simulink model "PlanerizerTest07_Flight_Stance"  (R2023a)
settings: Solver=FixedStepAuto  StartTime=0.0  StopTime=inf  FixedStep=0.005  RelTol=1e-3
libraries: canmsglib x8, speedgoatlib_IO691 x7, slrealtimeutilitieslib x3
settings Model: NumberOfSteps=2  ExtModeEnableFloating=off  Creator=celwe  LastModifiedBy=johna
settings SolverCC: ConcurrentTasks=on  PositivePriorityOrder=on
settings OptimizationCC: BlockReduction=off  OptimizeBlockIOStorage=off
settings DebuggingCC: TasksWithSamePriorityMsg=none  UnconnectedInputMsg=warning  UnconnectedOutputMsg=warning  UnconnectedLineMsg=warning
settings HardwareCC: ProdBitPerLong=64  ProdLongLongMode=on  ProdHWDeviceType=Intel->x86-64 (Linux 64)
settings ModelReferenceCC: EnableRefExpFcnMdlSchedulingChecks=on
settings RTWCC: Description=Simulink Real-Time  SystemTargetFile=slrealtime.tlc  TemplateMakefile=slrealtime_default_tmf  Toolchain=Simulink Real-Time Toolchain  BuildConfiguration=Faster Runs  CodeExecutionProfiling=on  TargetLang=C++  DLArmComputeVersion=19.05

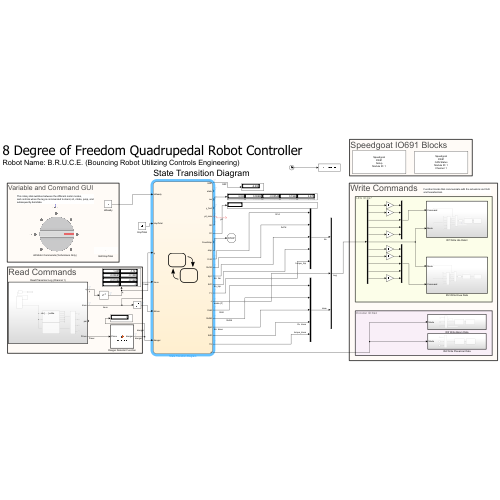
[thumbnail: Simulink's stored preview of the top-level diagram]
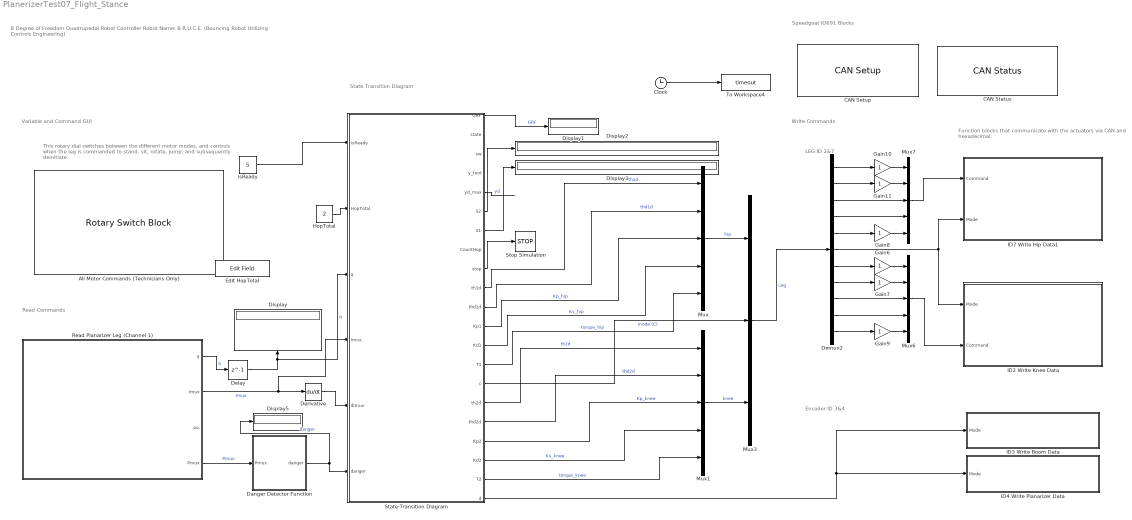
== system PlanerizerTest07_Flight_Stance ==
  note: Variable and Command GUI
  note: 8 Degree of Freedom Quadrupedal Robot Controller
      | Robot Name: B.R.U.C.E. (Bouncing Robot Utilizing Controls Engineering)
  note: This rotary dial switches between the different motor modes,
      | and controls when the leg is commanded to stand, sit, rotate, jump, and
      | subsequently deinitiate.
  note: LEG ID 2&7
  note: Function blocks that communicate with the actuators via CAN
      | and hexadecimal.
  note: Speedgoat IO691 Blocks
  note: Write Commands
  note: State Transition Diagram
  note: Encoder ID 3&4
  note: Read Commands
  "All Motor Commands (Technicians Only) " : RotarySwitchBlock
      settings: Values={{'Zeroing Planarizer', 'Zeroing Leg', 'Initiated', 'Control', 'deinit', 'Flight', 'test'}, [0 1 2 3 4 5 6]}
  "CAN Setup " : speedgoatlib_IO691/Legacy/CAN Setup   moduletype=IO691  id=1  pciSlot=-1  chn1=CAN (HS)  chn2=CAN (HS)  chn3=Disabled  chn4=Disabled  initStruct=[]  termStruct=[]  ArbitrationbdrChn1=1.0 MBaud  ArbitrationManbdrChn1=[2,8,31,8]  FdbdrChn1=5.0 MBaud  FdManbdrChn1=[2,2,5,2]  ArbitrationbdrChn2=1.0 MBaud  ArbitrationManbdrChn2=[2,8,31,8]  FdbdrChn2=5.0 MBaud  FdManbdrChn2=[2,2,5,2]  ArbitrationbdrChn3=1.0 MBaud  ArbitrationManbdrChn3=[2,8,31,8]  FdbdrChn3=5.0 MBaud  FdManbdrChn3=[2,2,5,2]  ArbitrationbdrChn4=1.0 MBaud  ArbitrationManbdrChn4=[2,8,31,8]  FdbdrChn4=5.0 MBaud  FdManbdrChn4=[2,2,5,2]  moduleInitValues=[691 1 -1 -1]
      settings: SourceProductName=Simulink Real-Time: Speedgoat I/O Blockset
  CAN Status : speedgoatlib_IO691/Legacy/CAN Status  moduleId=1  sampleTime=-1  channel=1  busRecovery=Off  arrayOutput=off  controllerCpuLoad=off  controllerLiveCount=off  initModeAct=off  avgBusLoad=off  receiving=off  RxQueueEmpty=off  dataOverrunRcv=off  rxBufferLevel=off  txPending=off  dataOverrunTx=off  txBufferLevel=off  errWarnLimit=off  errPassLimit=off  errBusOff=off  busRecoveryCounter=off  busCouplingErr=off  transceiverErr=off  opMode=off  brp=off  timeSegment1=off  timeSegment2=off  synchronisationJumpWidth=off  dataTSEG1=off  dataTSEG2=off  dataSJW=off  moduleType=691  qtyStatBlk=1  ptIdx=0  isFDMod=0
      settings: SourceProductName=Simulink Real-Time: Speedgoat I/O Blockset
  Clock : Clock
  Danger Detector Function : MATLAB Function  TreatAsAtomicUnit=on
  Delay : Delay  DelayLength=1
  Demux2 : Demux  Outputs=11
  Derivative : Derivative
  Display{,1..3,5} (5 alike) : Display
  Edit HopTotal : EditField  LabelPosition=Hide  ShowInitialText=on  Alignment=Center
  Gain{6..11} (6 alike) : Gain
  HopTotal : Constant  Value=2
  ID2 Write Knee Data : Subsystem  TreatAsAtomicUnit=on
  ID3 Write Boom Data : Subsystem  TreatAsAtomicUnit=on
  ID4 Write Planarizer Data : Subsystem  TreatAsAtomicUnit=on
  ID7 Write Hip Data1 : Subsystem  TreatAsAtomicUnit=on
  Mux{,1,6..7} (4 alike) : Mux  Inputs=5
  Mux3 : Mux  Inputs=3
  Read Planarizer Leg (Channel 1) : Subsystem  TreatAsAtomicUnit=on
  State-Transition Diagram : Stateflow chart  TreatAsAtomicUnit=on
      settings: PortSchema="{\"entries\":[{\"content\":{\"sides\":[{\"content\":{\"connectorIds\":[\"In3\",\"In5\",\"In1\",\"In6\",\"In4\",\"In2\"]},\"type\":\"ConnectorPlacement.EquallySpacedRectSide\",\"uuid\":\"09499f21-f50c-4ce4-914e-8b9942bcc246\"},{\"content\":{\"connectorIds\":[\"Out14\",\"Out16\",\"Out17\",\"Out18\",\"Out19\",\"Out20\",\"Out21\",\"Out15\",\"Out1\",\"Out10\",\"Out12\",\"Out5\",\"Out7\",\"Out3\",\"Out2\",\"Out11\",\"Out13\",\"Out6\",\"Out8\",\"Out4\",\"Out9\"],\"side\":\"RIGHT\"},\"type\":\"ConnectorPlacement.EquallySpacedRectSide\",\"uuid\":\"b935e908-ace3-4dfb-ad6d-08dfed6ffdb3\"},{\"content\":{\"side\":\"TOP\"},\"type\":\"ConnectorPlacement.EquallySpacedRectSide\",\"uuid\":\"4cd7c5d6-1f1f-4a1f-84b4-9b198395645e\"}]},\"type\":\"ConnectorPlacement.EquallySpacedConnector\",\"uuid\":\"2dc6a8af-05a8-4f21-87ab-6863f156f450\"}],\"packageUris\":[\"http://schema.mathworks.com/mf0/Connector/R2020b\"],\"version\":\"1.0\"}"
  Stop Simulation : Stop
  To Workspace4 : ToWorkspace  VariableName=timeout  SampleTime=-1
  isReady : Constant  Value=5
  wires:
  Mux/1 -> Mux3/1  "hip"
  State-Transition Diagram/3(T1) -> Mux/5  "torque_hip"
  Mux1/1 -> Mux3/3  "knee"
  State-Transition Diagram/2(c) -> Mux3/2  "mode (C)"
  isReady/1 -> State-Transition Diagram/3(isReady)
  Clock/1 -> To Workspace4/1
  Mux3/1 -> Demux2/1  "Leg"
  Mux7/1 -> ID7 Write Hip Data1/1(Command)
  Mux6/1 -> ID2 Write Knee Data/2(Command)
  Demux2/6 -> ID2 Write Knee Data/1(Mode), ID7 Write Hip Data1/2(Mode)
  Demux2/3 -> Mux7/3
  Demux2/8 -> Gain7/1
  Demux2/5 -> Gain8/1
  Demux2/4 -> Mux7/4
  Demux2/9 -> Mux6/3
  Demux2/2 -> Gain11/1
  Demux2/10 -> Mux6/4
  Gain11/1 -> Mux7/2
  Gain10/1 -> Mux7/1
  Gain7/1 -> Mux6/2
  Demux2/11 -> Gain9/1
  Gain9/1 -> Mux6/5
  Gain8/1 -> Mux7/5
  Gain6/1 -> Mux6/1
  State-Transition Diagram/8(Kd2) -> Mux1/4  "Kv_knee"
  State-Transition Diagram/4(T2) -> Mux1/5  "torque_knee"
  Demux2/1 -> Gain10/1
  Demux2/7 -> Gain6/1
  State-Transition Diagram/10(th1d) -> Mux/1  "th1d"
  State-Transition Diagram/12(thd1d) -> Mux/2  "thd1d"
  State-Transition Diagram/7(Kd1) -> Mux/4  "Kv_hip"
  State-Transition Diagram/5(Kp1) -> Mux/3  "Kp_hip"
  State-Transition Diagram/11(th2d) -> Mux1/1  "th2d"
  State-Transition Diagram/13(thd2d) -> Mux1/2  "thd2d"
  State-Transition Diagram/6(Kp2) -> Mux1/3  "Kp_knee"
  State-Transition Diagram/9(d) -> ID3 Write Boom Data/1(Mode), ID4 Write Planarizer Data/1(Mode)
  State-Transition Diagram/1(stop) -> Stop Simulation/1
  State-Transition Diagram/14(GRF) -> Display1/1  "GRF"
  Read Planarizer Leg (Channel 1)/2(Imux) -> State-Transition Diagram/6(Imux), Derivative/1  "Imux"
  Read Planarizer Leg (Channel 1)/1(q) -> Delay/1  "q"
  Delay/1 -> State-Transition Diagram/1(q), Display/1  "q"
  Danger Detector Function/1(danger) -> Display5/1, State-Transition Diagram/2(danger)  "danger"
  Derivative/1 -> State-Transition Diagram/4(dImux)
  Read Planarizer Leg (Channel 1)/4(Pmux) -> Danger Detector Function/1(Pmux)  "Pmux"
  HopTotal/1 -> State-Transition Diagram/5(HopTotal)
  State-Transition Diagram/19(yd_max) -> ?  "yd"
  State-Transition Diagram/20(S2) -> Display2/1
  State-Transition Diagram/21(S1) -> Display3/1

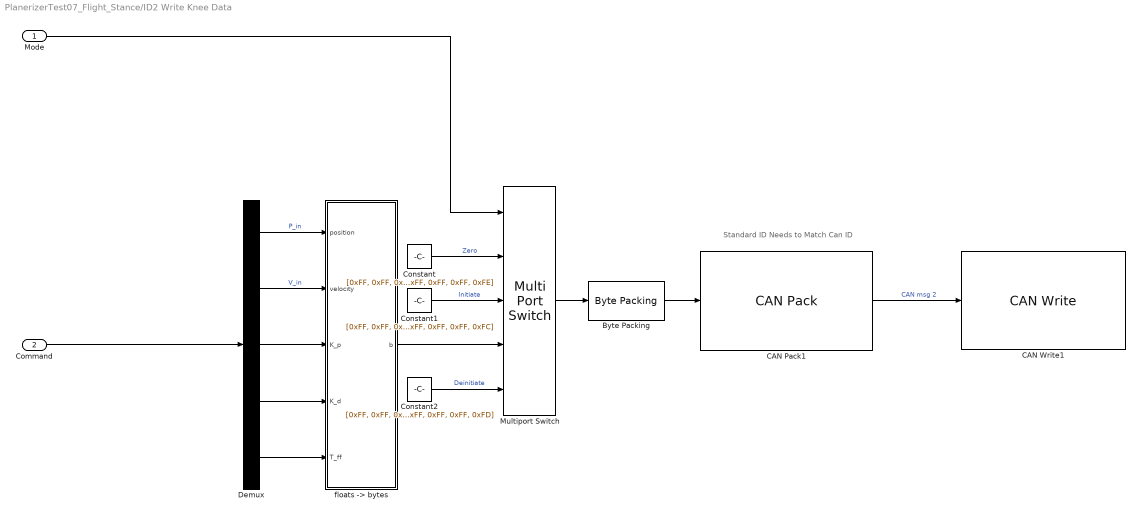
== system PlanerizerTest07_Flight_Stance/ID2 Write Knee Data ==
  note: Standard ID Needs to Match Can ID
  Mode : Inport
  Command : Inport  Port=2
  Byte Packing : slrealtimeutilitieslib/Byte Packing  MaskPackedDataType=uint8  MaskUnpackedDataTypes={['uint8']}  MaskAlignment=1
  CAN Pack1 : canmsglib/CAN Pack  MsgList=(none)  MsgName=CAN Msg  MsgIDType=Standard (11-bit identifier)  MsgIdentifier=2  MsgLength=8  Remote=off  ApplyMinMax=off  BusOutput=off  SignalInfo={ 'b1', '0', '8', 'LE', 'unsigned', 'Standard', '0', '1', '0', '-Inf', 'Inf'; 'b2', '8', '8', 'LE', 'unsigned', 'Standard', '0', '1', '0', '-Inf', 'Inf'; 'b3', '16', '8', 'LE', 'unsigned', 'Standard', '0', '1', '0', '-Inf', 'Inf'; 'b4', '24', '8', 'LE', 'unsigned', 'Standard', '0', '1', '0', '-Inf', 'Inf'; 'b5', '32', '8', 'LE', 'unsigned', 'Standard', '0', '1', '0', '-Inf', 'Inf'; 'b6', '40', '8', 'LE', 'unsigned', 'Standard', '0', '1', '0', '-Inf', 'Inf'; 'b7', '48', '8', 'LE', 'unsigned', 'Standard', '0', '1', '0', '-Inf', 'Inf'; 'b8', '56', '8', 'LE', 'unsigned', 'Standard', '0', '1', '0', '-Inf', 'Inf' }
      settings: DataFormat=raw data
  CAN Write1 : speedgoatlib_IO691/Legacy/CAN Write  id=1  ts=-1  channel=1  messageType=CAN  BusInput=off  enableStatusPort=off  canType=CAN (HS)  initValues=[691 1 -1 0 1 1 0 0]
      settings: SourceProductName=Simulink Real-Time: Speedgoat I/O Blockset
  Constant : Constant  Value=[0xFF, 0xFF, 0xFF, 0xFF, 0xFF, 0xFF, 0xFF, 0xFE]
  Constant1 : Constant  Value=[0xFF, 0xFF, 0xFF, 0xFF, 0xFF, 0xFF, 0xFF, 0xFC]
  Constant2 : Constant  Value=[0xFF, 0xFF, 0xFF, 0xFF, 0xFF, 0xFF, 0xFF, 0xFD]
  Demux : Demux  Outputs=5
  Multiport Switch : MultiPortSwitch  Inputs=4  DiagnosticForDefault=None  SaturateOnIntegerOverflow=off  InputSameDT=off
  "floats -> bytes" : MATLAB Function  TreatAsAtomicUnit=on
  wires:
  Demux/5 -> "floats -> bytes"/5(T_ff)
  Multiport Switch/1 -> Byte Packing/1
  Demux/4 -> "floats -> bytes"/4(K_d)
  Demux/1 -> "floats -> bytes"/1(position)  "P_in"
  Constant/1 -> Multiport Switch/2  "Zero"
  Demux/2 -> "floats -> bytes"/2(velocity)  "V_in"
  Constant2/1 -> Multiport Switch/5  "Deinitiate"
  CAN Pack1/1 -> CAN Write1/1  "CAN msg 2"
  Byte Packing/1 -> CAN Pack1/1
  Constant1/1 -> Multiport Switch/3  "Initiate"
  "floats -> bytes"/1(b) -> Multiport Switch/4
  Demux/3 -> "floats -> bytes"/3(K_p)
  Mode/1 -> Multiport Switch/1
  Command/1 -> Demux/1

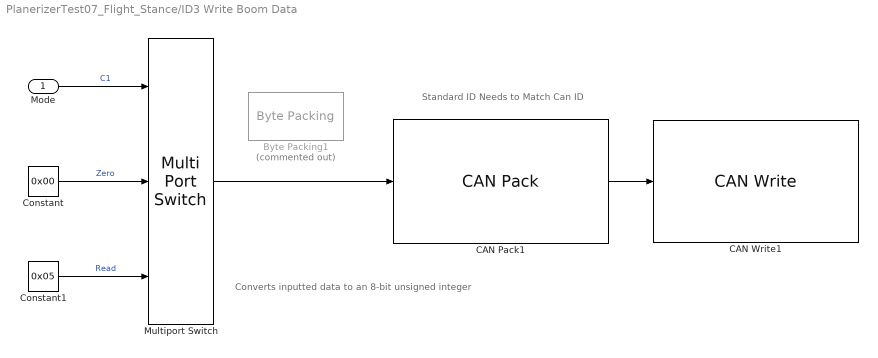
== system PlanerizerTest07_Flight_Stance/ID3 Write Boom Data ==
  note: Standard ID Needs to Match Can ID
  note: Converts inputted data to an 8-bit unsigned integer
  Mode : Inport
  Byte Packing1 : slrealtimeutilitieslib/Byte Packing  Commented=on  MaskPackedDataType=uint8  MaskUnpackedDataTypes={['uint8']}  MaskAlignment=1
  CAN Pack1 : canmsglib/CAN Pack  MsgList=(none)  MsgName=CAN Msg  MsgIDType=Standard (11-bit identifier)  MsgIdentifier=3  MsgLength=1  Remote=off  ApplyMinMax=off  BusOutput=off  SignalInfo={ 'b1', '0', '8', 'LE', 'unsigned', 'Standard', '0', '1', '0', '-Inf', 'Inf'; 'b2', '8', '8', 'LE', 'unsigned', 'Standard', '0', '1', '0', '-Inf', 'Inf'; 'b3', '16', '8', 'LE', 'unsigned', 'Standard', '0', '1', '0', '-Inf', 'Inf'; 'b4', '24', '8', 'LE', 'unsigned', 'Standard', '0', '1', '0', '-Inf', 'Inf'; 'b5', '32', '8', 'LE', 'unsigned', 'Standard', '0', '1', '0', '-Inf', 'Inf'; 'b6', '40', '8', 'LE', 'unsigned', 'Standard', '0', '1', '0', '-Inf', 'Inf'; 'b7', '48', '8', 'LE', 'unsigned', 'Standard', '0', '1', '0', '-Inf', 'Inf'; 'b8', '56', '8', 'LE', 'unsigned', 'Standard', '0', '1', '0', '-Inf', 'Inf' }
      settings: DataFormat=raw data
  CAN Write1 : speedgoatlib_IO691/Legacy/CAN Write  id=1  ts=-1  channel=1  messageType=CAN  BusInput=off  enableStatusPort=off  canType=CAN (HS)  initValues=[691 1 -1 0 1 1 0 0]
      settings: SourceProductName=Simulink Real-Time: Speedgoat I/O Blockset
  Constant : Constant  Value=0x00
  Constant1 : Constant  Value=0x05
  Multiport Switch : MultiPortSwitch  Inputs=2  DiagnosticForDefault=None  OutMin=0  SaturateOnIntegerOverflow=off  InputSameDT=off
  wires:
  Constant/1 -> Multiport Switch/2  "Zero"
  CAN Pack1/1 -> CAN Write1/1
  Multiport Switch/1 -> CAN Pack1/1
  Constant1/1 -> Multiport Switch/3  "Read"
  Mode/1 -> Multiport Switch/1  "C1"

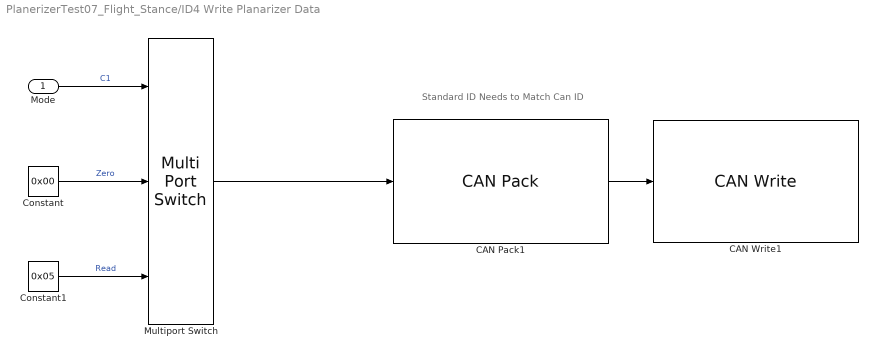
== system PlanerizerTest07_Flight_Stance/ID4 Write Planarizer Data ==
  note: Standard ID Needs to Match Can ID
  Mode : Inport
  CAN Pack1 : canmsglib/CAN Pack  MsgList=(none)  MsgName=CAN Msg  MsgIDType=Standard (11-bit identifier)  MsgIdentifier=4  MsgLength=1  Remote=off  ApplyMinMax=off  BusOutput=off  SignalInfo={ 'b1', '0', '8', 'LE', 'unsigned', 'Standard', '0', '1', '0', '-Inf', 'Inf'; 'b2', '8', '8', 'LE', 'unsigned', 'Standard', '0', '1', '0', '-Inf', 'Inf'; 'b3', '16', '8', 'LE', 'unsigned', 'Standard', '0', '1', '0', '-Inf', 'Inf'; 'b4', '24', '8', 'LE', 'unsigned', 'Standard', '0', '1', '0', '-Inf', 'Inf'; 'b5', '32', '8', 'LE', 'unsigned', 'Standard', '0', '1', '0', '-Inf', 'Inf'; 'b6', '40', '8', 'LE', 'unsigned', 'Standard', '0', '1', '0', '-Inf', 'Inf'; 'b7', '48', '8', 'LE', 'unsigned', 'Standard', '0', '1', '0', '-Inf', 'Inf'; 'b8', '56', '8', 'LE', 'unsigned', 'Standard', '0', '1', '0', '-Inf', 'Inf' }
      settings: DataFormat=raw data
  CAN Write1 : speedgoatlib_IO691/Legacy/CAN Write  id=1  ts=-1  channel=1  messageType=CAN  BusInput=off  enableStatusPort=off  canType=CAN (HS)  initValues=[691 1 -1 0 1 1 0 0]
      settings: SourceProductName=Simulink Real-Time: Speedgoat I/O Blockset
  Constant : Constant  Value=0x00
  Constant1 : Constant  Value=0x05
  Multiport Switch : MultiPortSwitch  Inputs=2  DiagnosticForDefault=None  SaturateOnIntegerOverflow=off  InputSameDT=off
  wires:
  Constant/1 -> Multiport Switch/2  "Zero"
  CAN Pack1/1 -> CAN Write1/1
  Multiport Switch/1 -> CAN Pack1/1
  Constant1/1 -> Multiport Switch/3  "Read"
  Mode/1 -> Multiport Switch/1  "C1"

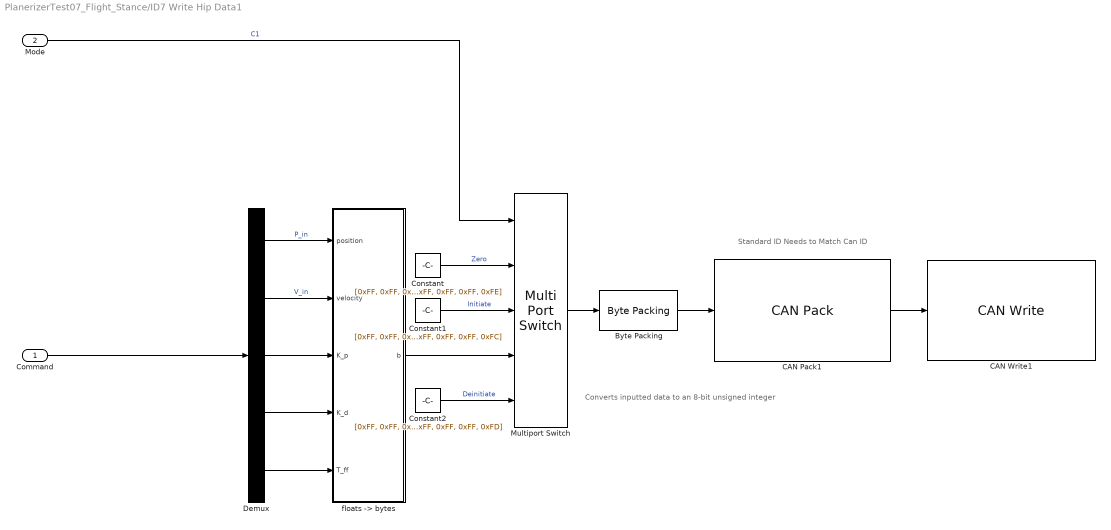
== system PlanerizerTest07_Flight_Stance/ID7 Write Hip Data1 ==
  note: Standard ID Needs to Match Can ID
  note: Converts inputted data to an 8-bit unsigned integer
  Command : Inport
  Mode : Inport  Port=2
  Byte Packing : slrealtimeutilitieslib/Byte Packing  MaskPackedDataType=uint8  MaskUnpackedDataTypes={['uint8']}  MaskAlignment=1
  CAN Pack1 : canmsglib/CAN Pack  MsgList=(none)  MsgName=CAN Msg  MsgIDType=Standard (11-bit identifier)  MsgIdentifier=7  MsgLength=8  Remote=off  ApplyMinMax=off  BusOutput=off  SignalInfo={ 'b1', '0', '8', 'LE', 'unsigned', 'Standard', '0', '1', '0', '-Inf', 'Inf'; 'b2', '8', '8', 'LE', 'unsigned', 'Standard', '0', '1', '0', '-Inf', 'Inf'; 'b3', '16', '8', 'LE', 'unsigned', 'Standard', '0', '1', '0', '-Inf', 'Inf'; 'b4', '24', '8', 'LE', 'unsigned', 'Standard', '0', '1', '0', '-Inf', 'Inf'; 'b5', '32', '8', 'LE', 'unsigned', 'Standard', '0', '1', '0', '-Inf', 'Inf'; 'b6', '40', '8', 'LE', 'unsigned', 'Standard', '0', '1', '0', '-Inf', 'Inf'; 'b7', '48', '8', 'LE', 'unsigned', 'Standard', '0', '1', '0', '-Inf', 'Inf'; 'b8', '56', '8', 'LE', 'unsigned', 'Standard', '0', '1', '0', '-Inf', 'Inf' }
      settings: DataFormat=raw data
  CAN Write1 : speedgoatlib_IO691/Legacy/CAN Write  id=1  ts=-1  channel=1  messageType=CAN  BusInput=off  enableStatusPort=off  canType=CAN (HS)  initValues=[691 1 -1 0 1 1 0 0]
      settings: SourceProductName=Simulink Real-Time: Speedgoat I/O Blockset
  Constant : Constant  Value=[0xFF, 0xFF, 0xFF, 0xFF, 0xFF, 0xFF, 0xFF, 0xFE]
  Constant1 : Constant  Value=[0xFF, 0xFF, 0xFF, 0xFF, 0xFF, 0xFF, 0xFF, 0xFC]
  Constant2 : Constant  Value=[0xFF, 0xFF, 0xFF, 0xFF, 0xFF, 0xFF, 0xFF, 0xFD]
  Demux : Demux  Outputs=5
  Multiport Switch : MultiPortSwitch  Inputs=4  DiagnosticForDefault=None  SaturateOnIntegerOverflow=off  InputSameDT=off
  "floats -> bytes" : MATLAB Function  TreatAsAtomicUnit=on
  wires:
  Demux/5 -> "floats -> bytes"/5(T_ff)
  Multiport Switch/1 -> Byte Packing/1
  Demux/4 -> "floats -> bytes"/4(K_d)
  Constant/1 -> Multiport Switch/2  "Zero"
  Demux/2 -> "floats -> bytes"/2(velocity)  "V_in"
  Constant2/1 -> Multiport Switch/5  "Deinitiate"
  CAN Pack1/1 -> CAN Write1/1
  Byte Packing/1 -> CAN Pack1/1
  Constant1/1 -> Multiport Switch/3  "Initiate"
  "floats -> bytes"/1(b) -> Multiport Switch/4
  Demux/3 -> "floats -> bytes"/3(K_p)
  Mode/1 -> Multiport Switch/1  "C1"
  Command/1 -> Demux/1
  Demux/1 -> "floats -> bytes"/1(position)  "P_in"

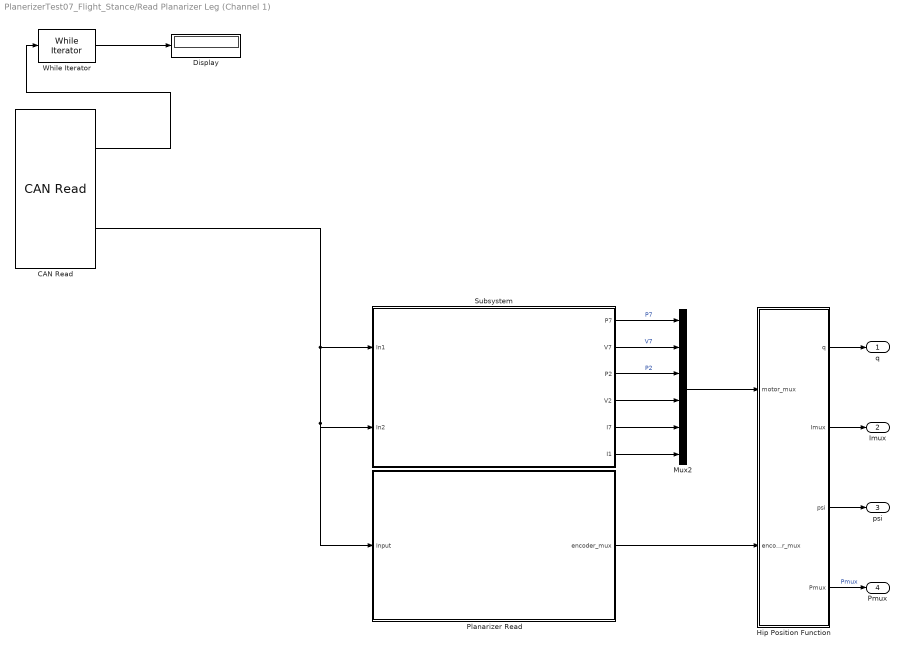
== system PlanerizerTest07_Flight_Stance/Read Planarizer Leg (Channel 1) ==
  CAN Read : speedgoatlib_IO691/Legacy/CAN Read  id=1  ts=-1  channel=1  messageType=CAN  canType=CAN (HS)  BusOutput=off  initValues=[691 1 -1 0 1 1 0]
      settings: SourceProductName=Simulink Real-Time: Speedgoat I/O Blockset
  Display : Display
  Hip Position Function : MATLAB Function  TreatAsAtomicUnit=on
  Mux2 : Mux  Inputs=6
  Planarizer Read : Subsystem
  Subsystem : Subsystem
  While Iterator : WhileIterator  MaxIters=-1  WhileBlockType=do-while  ResetStates=reset  ShowIterationPort=on
  q : Outport
  Imux : Outport  Port=2
  psi : Outport  Port=3
  Pmux : Outport  Port=4
  wires:
  CAN Read/1 -> While Iterator/1
  While Iterator/1 -> Display/1
  CAN Read/2 -> Planarizer Read/1(Input), Subsystem/2(In2), Subsystem/1(In1)
  Subsystem/1(P7) -> Mux2/1  "P7"
  Subsystem/3(P2) -> Mux2/3  "P2"
  Subsystem/2(V7) -> Mux2/2  "V7"
  Subsystem/4(V2) -> Mux2/4
  Planarizer Read/1(encoder_mux) -> Hip Position Function/2(encoder_mux)
  Mux2/1 -> Hip Position Function/1(motor_mux)
  Hip Position Function/1(q) -> q/1
  Hip Position Function/3(psi) -> psi/1
  Hip Position Function/4(Pmux) -> Pmux/1  "Pmux"
  Subsystem/5(I7) -> Mux2/5
  Subsystem/6(I1) -> Mux2/6
  Hip Position Function/2(Imux) -> Imux/1

== system PlanerizerTest07_Flight_Stance/Read Planarizer Leg (Channel 1)/Planarizer Read ==
  note: Encoder Read Command
  Input : Inport
  MATLAB Function : MATLAB Function  TreatAsAtomicUnit=on
  Mux : Mux
  Read Planarizer Leg (Chaannel 1) : Subsystem  TreatAsAtomicUnit=on
  encoder_mux : Outport
  wires:
  Read Planarizer Leg (Chaannel 1)/4(V4) -> Mux/4  "V4"
  Mux/1 -> MATLAB Function/1(in)
  Read Planarizer Leg (Chaannel 1)/1(P3) -> Mux/1  "P3"
  Read Planarizer Leg (Chaannel 1)/2(V3) -> Mux/2  "V3"
  Read Planarizer Leg (Chaannel 1)/3(P4) -> Mux/3  "P4"
  MATLAB Function/1(encoder_mux) -> encoder_mux/1
  Input/1 -> Read Planarizer Leg (Chaannel 1)/1(Input)

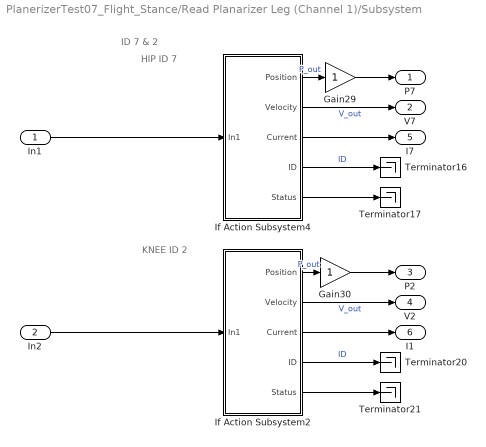
== system PlanerizerTest07_Flight_Stance/Read Planarizer Leg (Channel 1)/Subsystem ==
  note: KNEE ID 2
  note: HIP ID 7
  note: ID 7 & 2
  In1 : Inport
  In2 : Inport  Port=2
  Gain29 : Gain
  Gain30 : Gain
  If Action Subsystem2 : Subsystem  TreatAsAtomicUnit=on
  If Action Subsystem4 : Subsystem  TreatAsAtomicUnit=on
  Terminator{16..17,20..21} (4 alike) : Terminator
  P7 : Outport
  V7 : Outport  Port=2
  P2 : Outport  Port=3
  V2 : Outport  Port=4
  I7 : Outport  Port=5
  I1 : Outport  Port=6
  wires:
  If Action Subsystem4/4(ID) -> Terminator16/1  "ID"
  If Action Subsystem2/2(Velocity) -> V2/1  "V_out"
  If Action Subsystem2/5(Status) -> Terminator21/1
  If Action Subsystem4/2(Velocity) -> V7/1  "V_out"
  If Action Subsystem4/1(Position) -> Gain29/1  "P_out"
  If Action Subsystem4/3(Current) -> I7/1
  Gain30/1 -> P2/1
  If Action Subsystem2/4(ID) -> Terminator20/1  "ID"
  Gain29/1 -> P7/1
  If Action Subsystem4/5(Status) -> Terminator17/1
  If Action Subsystem2/1(Position) -> Gain30/1  "P_out"
  If Action Subsystem2/3(Current) -> I1/1
  In1/1 -> If Action Subsystem4/1(In1)
  In2/1 -> If Action Subsystem2/1(In1)

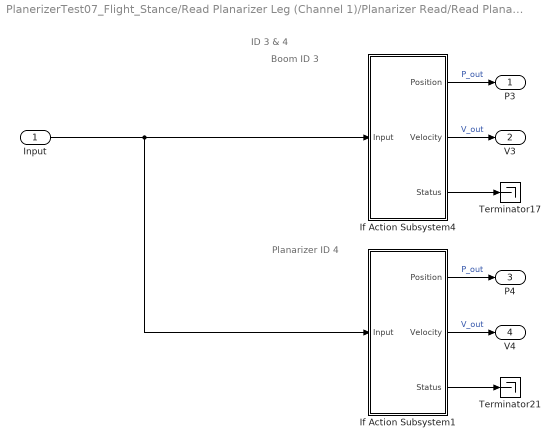
== system PlanerizerTest07_Flight_Stance/Read Planarizer Leg (Channel 1)/Planarizer Read/Read Planarizer Leg (Chaannel 1) ==
  note: Planarizer ID 4
  note: Boom ID 3
  note: ID 3 & 4
  Input : Inport
  If Action Subsystem1 : Subsystem  TreatAsAtomicUnit=on
  If Action Subsystem4 : Subsystem  TreatAsAtomicUnit=on
  Terminator17 : Terminator
  Terminator21 : Terminator
  P3 : Outport
  V3 : Outport  Port=2
  P4 : Outport  Port=3
  V4 : Outport  Port=4
  wires:
  If Action Subsystem1/1(Position) -> P4/1  "P_out"
  If Action Subsystem4/1(Position) -> P3/1  "P_out"
  If Action Subsystem4/3(Status) -> Terminator17/1
  If Action Subsystem1/2(Velocity) -> V4/1  "V_out"
  If Action Subsystem1/3(Status) -> Terminator21/1
  If Action Subsystem4/2(Velocity) -> V3/1  "V_out"
  Input/1 -> If Action Subsystem1/1(Input), If Action Subsystem4/1(Input)

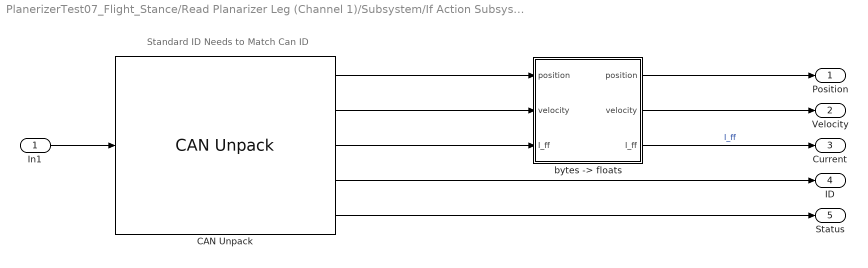
== system PlanerizerTest07_Flight_Stance/Read Planarizer Leg (Channel 1)/Subsystem/If Action Subsystem2 ==
  note: Standard ID Needs to Match Can ID
  In1 : Inport
  CAN Unpack : canmsglib/CAN Unpack  MsgList=(none)  MsgName=CAN Msg  MsgIDType=Standard (11-bit identifier)  MsgIdentifier=2  MsgLength=6  SignalInfo={ 'position', '16', '16', 'BE', 'unsigned', 'Standard', '0', '1', '0', '0', '65535'; 'velocity', '36', '12', 'BE', 'unsigned', 'Standard', '0', '1', '0', '0', '4095'; 'current', '40', '12', 'BE', 'unsigned', 'Standard', '0', '1', '0', '0', '4095'; 'id', '0', '8', 'BE', 'unsigned', 'Standard', '0', '1', '0', '0', '255' }  IDPort=off  TimestampPort=off  ErrorPort=off  RemotePort=off  LengthPort=off  StatusPort=on  ApplyMinMax=off
  "bytes -> floats" : MATLAB Function  TreatAsAtomicUnit=on
  Position : Outport
  Velocity : Outport  Port=2
  Current : Outport  Port=3
  ID : Outport  Port=4
  Status : Outport  Port=5
  wires:
  CAN Unpack/5 -> Status/1
  CAN Unpack/1 -> "bytes -> floats"/1("position ")
  CAN Unpack/3 -> "bytes -> floats"/3("I_ff ")
  "bytes -> floats"/1(position) -> Position/1
  CAN Unpack/4 -> ID/1
  "bytes -> floats"/2(velocity) -> Velocity/1
  "bytes -> floats"/3(I_ff) -> Current/1  "I_ff"
  CAN Unpack/2 -> "bytes -> floats"/2("velocity ")
  In1/1 -> CAN Unpack/1

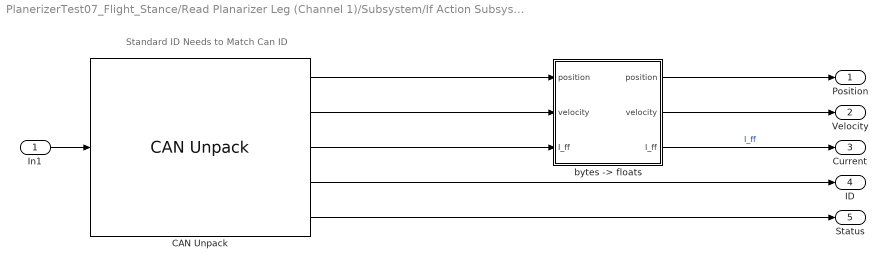
== system PlanerizerTest07_Flight_Stance/Read Planarizer Leg (Channel 1)/Subsystem/If Action Subsystem4 ==
  note: Standard ID Needs to Match Can ID
  In1 : Inport
  CAN Unpack : canmsglib/CAN Unpack  MsgList=(none)  MsgName=CAN Msg  MsgIDType=Standard (11-bit identifier)  MsgIdentifier=7  MsgLength=6  SignalInfo={ 'position', '16', '16', 'BE', 'unsigned', 'Standard', '0', '1', '0', '0', '65535'; 'velocity', '36', '12', 'BE', 'unsigned', 'Standard', '0', '1', '0', '0', '4095'; 'current', '40', '12', 'BE', 'unsigned', 'Standard', '0', '1', '0', '0', '4095'; 'id', '0', '8', 'BE', 'unsigned', 'Standard', '0', '1', '0', '0', '255' }  IDPort=off  TimestampPort=off  ErrorPort=off  RemotePort=off  LengthPort=off  StatusPort=on  ApplyMinMax=off
  "bytes -> floats" : MATLAB Function  TreatAsAtomicUnit=on
  Position : Outport
  Velocity : Outport  Port=2
  Current : Outport  Port=3
  ID : Outport  Port=4
  Status : Outport  Port=5
  wires:
  CAN Unpack/5 -> Status/1
  CAN Unpack/3 -> "bytes -> floats"/3("I_ff ")
  CAN Unpack/4 -> ID/1
  "bytes -> floats"/2(velocity) -> Velocity/1
  "bytes -> floats"/3(I_ff) -> Current/1  "I_ff"
  CAN Unpack/2 -> "bytes -> floats"/2("velocity ")
  In1/1 -> CAN Unpack/1
  CAN Unpack/1 -> "bytes -> floats"/1("position ")
  "bytes -> floats"/1(position) -> Position/1

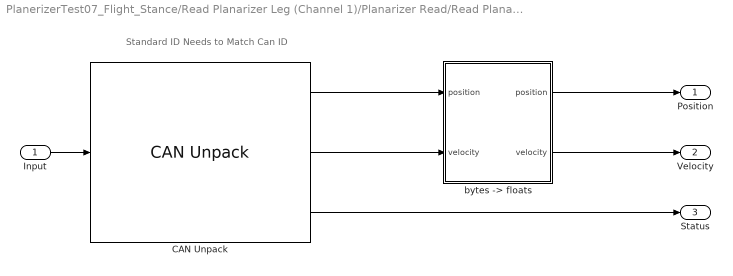
== system PlanerizerTest07_Flight_Stance/Read Planarizer Leg (Channel 1)/Planarizer Read/Read Planarizer Leg (Chaannel 1)/If Action Subsystem1 ==
  note: Standard ID Needs to Match Can ID
  Input : Inport
  CAN Unpack : canmsglib/CAN Unpack  MsgList=(none)  MsgName=CAN Msg  MsgIDType=Standard (11-bit identifier)  MsgIdentifier=4  MsgLength=6  SignalInfo={ 'position', '0', '32', 'LE', 'signed', 'Standard', '0', '1', '0', '0', '4294967295'; 'velocity', '32', '16', 'LE', 'signed', 'Standard', '0', '1', '0', '0', '65535' }  IDPort=off  TimestampPort=off  ErrorPort=off  RemotePort=off  LengthPort=off  StatusPort=on  ApplyMinMax=off
  "bytes -> floats" : MATLAB Function  TreatAsAtomicUnit=on
  Position : Outport
  Velocity : Outport  Port=2
  Status : Outport  Port=3
  wires:
  CAN Unpack/3 -> Status/1
  "bytes -> floats"/2(velocity) -> Velocity/1
  CAN Unpack/2 -> "bytes -> floats"/2("velocity ")
  Input/1 -> CAN Unpack/1
  CAN Unpack/1 -> "bytes -> floats"/1("position ")
  "bytes -> floats"/1(position) -> Position/1

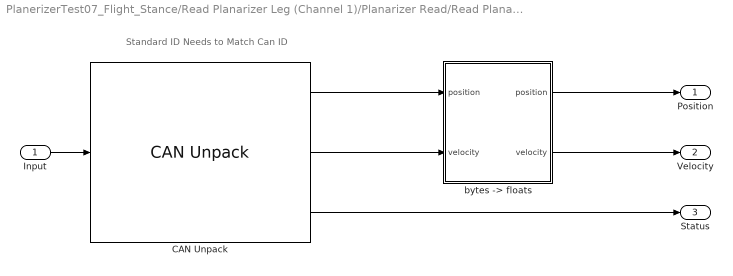
== system PlanerizerTest07_Flight_Stance/Read Planarizer Leg (Channel 1)/Planarizer Read/Read Planarizer Leg (Chaannel 1)/If Action Subsystem4 ==
  note: Standard ID Needs to Match Can ID
  Input : Inport
  CAN Unpack : canmsglib/CAN Unpack  MsgList=(none)  MsgName=CAN Msg  MsgIDType=Standard (11-bit identifier)  MsgIdentifier=3  MsgLength=6  SignalInfo={ 'position', '0', '32', 'LE', 'signed', 'Standard', '0', '1', '0', '0', '4294967295'; 'velocity', '32', '16', 'LE', 'signed', 'Standard', '0', '1', '0', '0', '65535' }  IDPort=off  TimestampPort=off  ErrorPort=off  RemotePort=off  LengthPort=off  StatusPort=on  ApplyMinMax=off
  "bytes -> floats" : MATLAB Function  TreatAsAtomicUnit=on
  Position : Outport
  Velocity : Outport  Port=2
  Status : Outport  Port=3
  wires:
  CAN Unpack/3 -> Status/1
  "bytes -> floats"/2(velocity) -> Velocity/1
  CAN Unpack/2 -> "bytes -> floats"/2("velocity ")
  Input/1 -> CAN Unpack/1
  CAN Unpack/1 -> "bytes -> floats"/1("position ")
  "bytes -> floats"/1(position) -> Position/1

== matlab function PlanerizerTest07_Flight_Stance/Read Planarizer Leg (Channel 1)/Subsystem/If Action Subsystem4/bytes -> floats ==
  data: position input; position output; velocity output; I_ff output; velocity input; I_ff input
function [position, velocity, I_ff] = fcn(position, velocity, I_ff)

P_MIN  =-95.5;  % [rad]
P_MAX  = 95.5;  % [rad]
V_MIN  =-45;    % [rad/s]
V_MAX  = 45;    % [rad/s]
I_MIN  =-40;    % []
I_MAX  = 40;    % []

position = position*(P_MAX  - P_MIN)/65535+ P_MIN;
velocity = velocity*(V_MAX  - V_MIN)/4095 + V_MIN;
I_ff     = I_ff*(I_MAX  - I_MIN)/4095 + I_MIN;

== matlab function PlanerizerTest07_Flight_Stance/Read Planarizer Leg (Channel 1)/Subsystem/If Action Subsystem2/bytes -> floats ==
  data: position input; position output; velocity output; I_ff output; velocity input; I_ff input
function [position, velocity, I_ff] = fcn(position, velocity, I_ff)

P_MIN  =-95.5;  % [rad]
P_MAX  = 95.5;  % [rad]
V_MIN  =-45;    % [rad/s]
V_MAX  = 45;    % [rad/s]
I_MIN  =-40;    % []
I_MAX  = 40;    % []

position = position*(P_MAX  - P_MIN)/65535+ P_MIN;
velocity = velocity*(V_MAX  - V_MIN)/4095 + V_MIN;
I_ff     = I_ff*(I_MAX  - I_MIN)/4095 + I_MIN;

== matlab function PlanerizerTest07_Flight_Stance/ID7 Write Hip Data1/floats -> bytes ==
  data: position input; b output uint8 size=8; velocity input; K_p input; K_d input; T_ff input
function b = fcn(position, velocity, K_p, K_d, T_ff)

P_MIN  =-95.5;  % [rad]
P_MAX  = 95.5;  % [rad]
V_MIN  =-45;    % [rad/s] 30 to 45
V_MAX  = 45;    % [rad/s]
KP_MIN = 0;     % [Nm/rad]
KP_MAX = 500;   % [Nm/rad]
KD_MIN = 0;     % [Nm*s/rad
KD_MAX = 5;     % [Nm*s/rad
T_MIN  =-18;    % [Nm]
T_MAX  = 18;    % [Nm]

position = floor((max(min(position,P_MAX) ,P_MIN)  - P_MIN )*65535/(P_MAX  - P_MIN));
velocity = floor((max(min(velocity,V_MAX) ,V_MIN)  - V_MIN )*4095 /(V_MAX  - V_MIN));
K_p      = floor((max(min(K_p     ,KP_MAX),KP_MIN) - KP_MIN)*4095 /(KP_MAX - KP_MIN));
K_d      = floor((max(min(K_d     ,V_MAX) ,V_MIN)  - KD_MIN)*4095 /(KD_MAX - KD_MIN));
T_ff     = floor((max(min(T_ff    ,V_MAX) ,V_MIN)  - T_MIN )*4095 /(T_MAX  - T_MIN));

p  = dec2bin(position);
p  = [repmat('0', 1, 16-length(p)),p];
v  = dec2bin(velocity);
v  = [repmat('0', 1, 12-length(v)),v];
kp = dec2bin(K_p);
kp  = [repmat('0', 1, 12-length(kp)),kp];
kd = dec2bin(K_d);
kd  = [repmat('0', 1, 12-length(kd)),kd];
t  = dec2bin(T_ff);
t  = [repmat('0', 1, 12-length(t)),t];

B = repmat('0', 8, 8);

B(1,:) = p(1:8);
B(2,:) = p(9:16);
B(3,:) = v(1:8);
B(4,:) = [v(9:12),kp(1:4)];
B(5,:) = kp(5:12);
B(6,:) = kd(1:8);
B(7,:) = [kd(9:12),t(1:4)];
B(8,:) = t(5:12);

B  = bin2dec(B);

b = uint8(B);

== matlab function PlanerizerTest07_Flight_Stance/Danger Detector Function ==
  data: Pmux input; danger output
function danger = isDanger(Pmux)
    % Pmux position matrix radians
    %       [p(ID1),p(ID2),p(ID3),p(IDN)]

        
    p1Max = 2; 
    p1Min = -2;
    p2Max = 2;
    p2Min = -2;
    
    P1 = Pmux(1:2:end);
    P2 = Pmux(2:2:end);
    
    danger = 0;
    if((0<sum((P1>p1Max) + (P1<p1Min))) || (0<sum((P2>p2Max) + (P2<p2Min))))
        danger = 1;
    end
end

== matlab function PlanerizerTest07_Flight_Stance/Read Planarizer Leg (Channel 1)/Planarizer Read/MATLAB Function ==
  data: in input; encoder_mux output
function encoder_mux = Pol2Cart(in)

% Variables
phi         = in(1);    % Boom Angle
phi_dot     = in(2);    % Boom Angular Velcoity
psi         = in(3);    % Planarizer Angle
psi_dot     = in(4);    % Planarizer Angular Velcoity

% Parameters
h           = .445;    % vertical height of base in meters
phi_offset  = .1995;        % Boom angle zero offset
b           = 1.2573;   % Length of boom to hip
e           = 0.137;    % horizantal length of encoders to mid-plane

% Outputs
x_hip = (e+b)*-psi;
x_dot_hip = (e+b)*-psi_dot;
y_hip = h - b*sin(phi+phi_offset);
y_dot_hip = - b*cos(phi+phi_offset)*phi_dot; 

encoder_mux = [x_hip x_dot_hip y_hip y_dot_hip psi];

== stateflow chart PlanerizerTest07_Flight_Stance/State-Transition Diagram ==
  state Start
  note: Simulink State Transition Diagram
      | "IsReady" is a user defined varable that controls the flow through the Finite State Mechine
      | Motor Commands: 1. Zero
      | (c) 2. Init
      | 3. Command
      | 4. Deinit
      | Encoder Commands: 1. Zero
      | (d) 2. Read
  state SlowDown
    entry:
    %deinitiate mode
    c = 4;
    d = 2;
  state ZeroPlanarizer
    entry:
    d = 1;
  state Init
    entry:
    c = 2;
    d = 2;
  state ZeroLeg
    entry:
    c = 1;
    to = 10;
  state Command
    entry:
    c = 3;
    tstep = 1.5;
    G = 1;
    n = 3;
    during:
    Tcalc1 = getT(Imux(1),q(1));
    Tcalc2 = getT(Imux(2),q(1)+q(2));
    [GRF,calcForceX] = getF(q,Tcalc1,Tcalc2);
    yd_filter  = AVGFilter(yd_filter,q(8),n);
    [y_foot,yd_foot] = getFootState(q,yd_filter);
    state Control [parallel]
      settings: executionOrder=1
      state ControllerSetup
        entry:
        %Flight
        sp = [.72 -1.15;0 0];
        Kp_f = [35,25];
        Kd_f = [50,10];
        F_offset = 1;
        %Stance
        w = 15*pi;
        Fxd = 0;
        yhipd = yhipCalc(sp,.5);
        Kp_s = [3; -3];
        Kdx_s = [-.12; .2];
        Kdy_s = [.05; -.1];
        % Temp Values
        Kp_temp = 30;
        Kd_temp = .2;
        %Goals
        th_LiftOff = deg2rad(65);
        Vxhipd = 1.5;
        offset = .5;
        Vyhipd = Vxhipd*tan(th_LiftOff);
      state Stand
        entry:
        state = 0;
        %Temp Gains
        Kp1 = Kp_temp;
        Kp2 = Kp_temp;
        Kd1 = Kd_temp;
        Kd2 = Kd_temp;
        %Stand Function
        to = t;
        th1d = q(1);
        tho1 = th1d;
        slope1 = (sp(1,1)*G - tho1)/tstep;
        th2d = q(2);
        tho2 = th2d;
        slope2 = (sp(1,2)*G - tho2)/tstep;
        during:
        th1d  = tho1  + slope1*(t-to);
        th2d  = tho2  + slope2*(t-to);
      state Ready2Jump
      state Airborn
        exit:
      state Stance
        during:
        T_ff = FeedForwardTorque(q,w,A,phi,Fxd,t-to);
        [T1, T2,S1,S2] = ControllerStance(q,Kp_s,Kdx_s,Kdy_s,T_ff,yhipd,Vxhipd,Vyhipd);
        exit:
        %Zeroing Torques
        T1 = 0;
        T2 = 0;
      state Transition2Stance
        entry:
        state = -2;
        to = t;
        %Stance Gains
        Kp1 = 0;
        Kp2 = 0;
        Kd1 = 0;
        Kd2 = 0;
        %Stance Transition
        [A,phi] = APhiGRFCalc(q,w,Vyhipd,GRF,F_offset)
      state Idle_Flight
        entry:
        state = 1
        idle = 0;
      state Flight
        during:
        [th1d,th2d,thd1d,thd2d] = Traj(t-to,tf,C);
        exit:
        % Zeroing Derivatives
        thd1d = 0;
        thd2d = 0;
        Kd1 = Kd_temp;
        Kd2 = Kd_temp;
      state Transition2Flight
        entry:
        state = 2;
        to = t;
        %Flight Gains
        Kp1 = Kp_f(1);
        Kp2 = Kp_f(2);
        Kd1 = Kd_f(1);
        Kd2 = Kd_f(2);
        %Flight Transition
        sp = Calc_Setpoint_Velcoity(q,sp,Vxhipd,offset);
        tf = FlightTimeApprox(y_max,yd_max,sp);
        C = TrajPlan(q,tf,sp);
        [th1d,th2d,thd1d,thd2d] = Traj(t-to,tf,C);
      state Idle_Stance
        entry:
        idle = 0;
      (default) -> ControllerSetup
      ControllerSetup -> Stand : {idle = 0;}
      Stand -> Ready2Jump : [(th1d >= sp(1,1)*G & slope1>0) | (th1d <= sp(1,1)*G & slope1<0)]
          | {th1d = sp(1,1)*G; th2d = sp(1,2)*G;}
      Ready2Jump -> Airborn : [isReady == 5 & sw == 0]
      Idle_Flight -> Stand [order 1] : [(isReady ~= 5 | CountHop >= HopTotal)]
      Airborn -> Transition2Stance : [after(2,sec)]
          | {CountHop = 0;}
      Idle_Flight -> Transition2Stance [order 2] : [sw == 0]
      Flight -> Idle_Flight : [after(tf,sec)]
      Transition2Stance -> Stance
      Transition2Flight -> Flight
      Idle_Stance -> Transition2Flight : [sw == 1]
      Stance -> Idle_Stance : [after(pi/w,sec)]
          | {CountHop = CountHop + 1;}
    state Detect [parallel]
      settings: executionOrder=2
      state Detect_Idle
        entry:
        idle = 1;
      state DetectImpact
        entry:
        I_lim =200*yd_max/.35;
        %I_sign1 = -q(1)/abs(q(1));
        %I_sign2 = -(q(1) + q(2))/abs(q(1) + q(2));
      state DetectLiftOff
        entry:
        yd_max = yd_filter;
      Detect_Idle -> DetectImpact [order 1] : [sw == 1 & idle == 0]
      DetectImpact -> Detect_Idle : [(abs(dImux(1)) > I_lim) | (abs(dImux(2)) > I_lim)]
          | {sw = 0;}
      (default) -> Detect_Idle : {sw = 1;}
      DetectLiftOff -> DetectLiftOff [order 2] : [yd_filter > yd_max]
      Detect_Idle -> DetectLiftOff [order 2] : [sw ==  0 & idle == 0]
      DetectLiftOff -> Detect_Idle [order 1] : [yd_max - yd_filter > .2]
          | {y_max = HipHeightAngleCalc(q); sw = 1;}
  state FinalShutdown
    entry:
    Kp1 = 0;
    Kp2 = 0;
    th1d = 0;
    th2d = 0;
    thd1d = 0;
    thd2d = 0;
    T1 = 0;
    T2 = 0;
    Kd1 = .1;
    Kd2 = .1;
  state Deinitiate
    entry:
    c = 4;
  (default) -> Start
  Start -> Init [order 2] : [isReady == 2]
  Start -> ZeroPlanarizer [order 1] : [isReady == 0 | isReady == 1]{to = 0;}
  SlowDown -> ZeroPlanarizer [order 2] : [after(.1,sec) & isReady == 0]
  ZeroPlanarizer -> SlowDown
  SlowDown -> Init [order 3] : [(isReady == 2 & to == 10) | isReady == 4]
  Init -> SlowDown [order 3] : [isReady == 0 | isReady == 1]
  Init -> FinalShutdown [order 2] : [isReady == 4 | danger == 1]
  Init -> Command [order 1] : [isReady == 3]
  ZeroLeg -> SlowDown
  SlowDown -> ZeroLeg [order 1] : [after(.5,sec) & isReady == 1 & ~(q(1) == q(2)) ]
  Command -> FinalShutdown : [isReady == 4 | danger == 1]
  FinalShutdown -> Deinitiate
  Deinitiate -> (junction 36) : after(3,sec)
  (junction 36) -> Deinitiate : {stop = 1;}
  data: YHIPD function_output; SP function_input; P function_input; A_Mag function_output; u function_input; W function_input; VYHIPD function_input; grf function_input; PHI function_output; OFFSET function_input; u function_input; SP function_output; SP function_input; VXHIPD function_input; OFFSET function_input; Y function_input; YD function_input; SP function_input; TF function_output; u function_input; TF function_input; SP function_input; C_mat function_output; TAU_ff function_output; u function_input; W function_input; A_Mag function_input; PHI function_input; FXD function_input; t function_input; t function_input; TF function_input; C_mat function_input; TH1D function_output; TH2D function_output; THD1D function_output; THD2D function_output; tau1 function_output double; u function_input; KP_s function_input; KDx_s function_input; KDy_s function_input; tau_ff function_input; YHIPd function_input; VXHIPd function_input; VYHIPd function_input; tau2 function_output; s1 function_output; s2 function_output; I function_input; CALC_T function_output; TH function_input; u function_input; T1CALC function_input; T2CALC function_input; calcFY function_output; calcFX function_output; in function_input; New function_input; out function_output; N function_input; u function_input; posy function_output; vely function_output; yd function_input; Y function_output; u function_input; q input; stop output =0; c output; T1 output =0; T2 output =0; Kp1 output =30; Kp2 output =30; Kd1 output =.2; Kd2 output =.2; danger input; isReady input; d output; th1d output =0; th2d output =0; thd1d output =0; thd2d output =0; Kd_f local; Kp_f local; Kp_s local; Vyhipd local; w local; Kd_temp local; Kp_temp local; Vxhipd local; to local; tho1 local; slope2 local; tho2 local; offset local; sp local; thd local; GRF output =0; calcForceX local; Tcalc1 local; Tcalc2 local; tstep local; slope1 local; th_LiftOff local; A local; CountHop output; Fxd local; T_ff local; phi local; yhipd local; tf local; C local; n local; G local; Kdx_s local; Kdy_s local; dImux input; state output; F_offset local; I_lim local; I_sign1 local; I_sign2 local; idle local; sw output; HopTotal input; yd_foot local; yd_filter local =0; y_foot output =0; y_max local; yd_max output; Imux input; S2 output; S1 output
  function YHIPD  = yhipCalc(SP,P):
    | function YHIPD  = yhipCalc(SP,P)
    | 
    |     % Length Constants
    |     LA = 0.1362;
    |     LB = 0.1636;
    | 
    |     YHIPD = (LB + LA)*(1-P) + (LA*cos(SP(1,1)) + LB*cos(SP(1,1)+SP(1,2)))*P;
    | end
  function [A_Mag,PHI] = APhiGRFCalc(u,W,VYHIPD,grf,OFFSET):
    | function [A_Mag,PHI] = APhiGRFCalc(u,W,VYHIPD,grf,OFFSET)
    | 
    |     % Mass Constants
    |     m0 = 0.665;
    |     m1 = 1.019;
    |     m2 = 0.128;
    |     % Length Constants
    |     LA = 0.1362;
    |     LB = 0.1636;
    | 
    | 
    |     %Actual hip velocity
    |     YD = u(5)*(-LB*sin(u(1)+u(2)) - LA*sin(u(1))) + u(6)*(-LB*sin(u(1)+u(2)));
    | 
    |     if grf > 800
    |         grf = 800;
    |     elseif grf < -800
    |         grf = -800;
    |     end
    |     
    |     A_Mag = OFFSET*(((m0+m1+m2)*W*(VYHIPD - YD))^2 + (grf)^2)/(2*(m0+m1+m2)*W*(VYHIPD - YD));
    |     PHI = asin(grf/A_Mag);
    | end
  function SP = Calc_Setpoint_Velcoity(u,SP,VXHIPD,OFFSET):
    | function SP = Calc_Setpoint_Velcoity(u,SP,VXHIPD,OFFSET)
    | 
    |     % Length Constants
    |     LA = 0.1362;
    |     LB = 0.1636;
    | 
    | 
    | 
    |     % CALC VX_FOOT
    |     VX_FOOT = u(7) + u(5)*LA*cos(u(1)) + (u(5)+ u(6))*LB*cos(u(1)+ u(2));
    | 
    |     % CALC NEW SETPOINT VELOCITY
    |     SP(2,1) = -2*(VXHIPD-VX_FOOT)*OFFSET/(LA*cos(SP(1,1)) + LB*cos(SP(1,1) + SP(1,2)));
    |     SP(2,2) = (VXHIPD-VX_FOOT)*OFFSET/(LB*cos(SP(1,1) + SP(1,2)));
    | end
  function TF = FlightTimeApprox(Y,YD,SP):
    | function TF = FlightTimeApprox(Y,YD,SP)
    | 
    |     % Mass Constants
    |     m0 = 0.665;
    |     m1 = 1.019;
    |     m2 = 0.128;
    |     % Length Constants
    |     LA = 0.1362;
    |     LB = 0.1636;
    |     L1 = 0.011;
    |     L2 = 0.0527;
    |     % Bar Mass Inertias
    |     I1 = 0.00207;
    |     I2 = 0.00191;
    |     % Damping Coefficents
    |     c1 = 0.00749;
    |     c2 = 1;
    |     % Gravity
    |     g = 7;
    | 
    |     yf = LA*cos(SP(1,1)) + LB*cos(SP(1,1)+SP(1,2));
    |     if((YD^2-2*g*(yf-Y))>=0)
    |         TF = (YD + sqrt(YD^2-2*g*(yf-Y)))/g;
    |     else
    |         TF = 0.005;
    |     end
    | end
  function C_mat = TrajPlan(u,TF,SP):
    | function C_mat = TrajPlan(u,TF,SP)
    | 
    |     M_t =[1   0    0    0;
    |           0   1    0    0;
    |           1   TF   TF^2 TF^3;
    |           0   1    2*TF 3*TF^2];
    | 
    |     M_IC = [u(1) u(2); u(5) u(6); SP];
    | 
    |     C_mat = M_t\M_IC;
    | end
  function TAU_ff  = FeedForwardTorque(u,W,A_Mag,PHI,FXD,t):
    | function TAU_ff  = FeedForwardTorque(u,W,A_Mag,PHI,FXD,t)
    | 
    |     % Mass Constants
    |     m0 = 0.665;
    |     m1 = 1.019;
    |     m2 = 0.128;
    |     % Length Constants
    |     LA = 0.1362;
    |     LB = 0.1636;
    |     L1 = 0.011;
    |     L2 = 0.0527;
    |     % Bar Mass Inertias
    |     I1 = 0.00207;
    |     I2 = 0.00191;
    |     % Damping Coefficents
    |     c1 = 0.00749;
    |     c2 = 1;
    |     % Gravity
    |     g = 9.81;
    | 
    |     Fd = [FXD; A_Mag*sin(W*t + PHI)];
    |     J = [LB*cos(u(1)+u(2)) + LA*cos(u(1))  LB*cos(u(1)+u(2));
    |         LB*sin(u(1)+u(2)) + LA*sin(u(1))  LB*sin(u(1)+u(2))];
    |     
    |     tau_mass = [m1*g*L1*sin(u(1)) + m2*g*(L2*sin(u(1)+u(2)) + LA*sin(u(1)));
    |               m2*g*L2*sin(u(1)+u(2))];
    |     TAU_ff = -J'*Fd + tau_mass;
    | end
  function [TH1D,TH2D,THD1D,THD2D] = Traj(t,TF,C_mat):
    | function [TH1D,TH2D,THD1D,THD2D] = Traj(t,TF,C_mat)
    | 
    |     if TF < t
    |         t = TF;
    |     end
    |     
    |     thd = [1 t   t^2 t^3;
    |            0 1 2*t 3*t^2]*C_mat;
    | 
    |     % Position th1d
    |     TH1D = thd(1,1);
    |     % Position th2d
    |     TH2D = thd(1,2);
    |     if TH2D < -1.8
    |         TH2D = -1.8;
    |     end
    |     % Position Derivative thd1d
    |     THD1D = thd(2,1);
    |     % Position Derivative thd2d
    |     THD2D = thd(2,2);
    | end
  function [tau1,tau2,s1,s2] = ControllerStance(u,KP_s,KDx_s,KDy_s,tau_ff,YHIPd,VXHIPd,VYHIPd):
    | function [tau1,tau2,s1,s2] = ControllerStance(u,KP_s,KDx_s,KDy_s,tau_ff,YHIPd,VXHIPd,VYHIPd)
    |     % Length Constants
    |     LA = 0.1362;
    |     LB = 0.1636;
    | 
    |     %Calculate Actual Values
    |     YHIPa = LB*cos(u(1)+u(2)) + LA*cos(u(1));
    |     VXHIPa = u(5)*(-LB*cos(u(1)+u(2)) - LA*cos(u(1))) + u(6)*(-LB*cos(u(1)+u(2)));
    |     VYHIPa = u(5)*(-LB*sin(u(1)+u(2)) - LA*sin(u(1))) + u(6)*(-LB*sin(u(1)+u(2)));
    | 
    |     % Hip y Position
    |     e_y = YHIPd - YHIPa;
    |     % Hip x Velecity
    |     e_Vx = VXHIPd - VXHIPa;
    |     % Hip y Velecity
    |     e_Vy = VYHIPd -VYHIPa;
    |     % Compute error Matricies
    | 
    |     T = tau_ff + KP_s*e_y + KDx_s*e_Vx + KDy_s*e_Vy;
    |     tau1 = T(1);
    |     tau2 = T(2);
    | 
    |     s1 = [tau_ff(1) KP_s(1)*e_y KDx_s(1)*e_Vx KDy_s(1)*e_Vy tau1];
    |     s2 = [tau_ff(2) KP_s(2)*e_y KDx_s(2)*e_Vx KDy_s(2)*e_Vy tau2];
    | end
  function CALC_T = getT(I,TH):
    | function CALC_T = getT(I,TH)
    |     CALC_T = I/abs(4.8*sin(TH));
    | end
  function [calcFY,calcFX] = getF(u,T1CALC,T2CALC):
    | function [calcFY,calcFX] = getF(u,T1CALC,T2CALC)
    | 
    |     % Length Constants
    |     LA = 0.1362;
    |     LB = 0.1636;
    | 
    | 
    |     J = [LB*cos(u(1)+u(2)) + LA*cos(u(1))  LB*cos(u(1)+u(2));
    |          LB*sin(u(1)+u(2)) + LA*sin(u(1))  LB*sin(u(1)+u(2))];
    |     %T_mass = [m1*g*L1*sin(u(1)) + m2*g*(L2*sin(u(1)+u(2)) + LA*sin(u(1)));
    |     %             m2*g*L2*sin(u(1)+u(2))]*0;
    | 
    |     T = [T1CALC;T2CALC];
    |     
    |     F = (-J')\(T); %check sign on T_mass
    | 
    |     calcFY = F(2);
    |     calcFX = F(1);
    | end
  function out  = AVGFilter(in,New,N):
    | function out  = AVGFilter(in,New,N)
    |     out = in*(N-1)/N+New/N;
    | end
  function [posy,vely]   = getFootState(u,yd):
    | function [posy,vely]   = getFootState(u,yd)
    |     % Length Constants
    |     LA = 0.1362;
    |     LB = 0.1636;
    | 
    |     r_foot = .055;
    | 
    | 
    |     x_foot = [u(3) + LA*sin(u(1)) + (LB-r_foot)*sin(u(1)+ u(2));
    |               u(4) - LA*cos(u(1)) - (LB-r_foot)*cos(u(1)+ u(2)) - r_foot];
    | 
    |     v_foot = [u(7) + u(5)*LA*cos(u(1)) + (u(5)+ u(6))*(LB-r_foot)*cos(u(1)+ u(2));
    |                 yd + u(5)*LA*sin(u(1)) + (u(5)+ u(6))*(LB-r_foot)*sin(u(1)+ u(2))];
    | 
    |     posy = x_foot(2);
    |     vely = v_foot(2);
    | end
  function Y   = HipHeightAngleCalc(u):
    | function Y   = HipHeightAngleCalc(u)
    |     % Length Constants
    |     LA = 0.1362;
    |     LB = 0.1636;
    | 
    | 
    |     Y = LB*cos(u(1)+u(2)) + LA*cos(u(1));
    |     %YD = u(5)*(-LB*sin(u(1)+u(2)) - LA*sin(u(1))) + u(6)*(-LB*sin(u(1)+u(2)));
    | end

== matlab function PlanerizerTest07_Flight_Stance/Read Planarizer Leg (Channel 1)/Hip Position Function ==
  data: q output; Imux output; psi output; motor_mux input; Pmux output; encoder_mux input
function [q,Imux,psi,Pmux] = Hip_Position(motor_mux,encoder_mux)
    q = [motor_mux(1),motor_mux(3),encoder_mux(1),encoder_mux(3),motor_mux(2),motor_mux(4),encoder_mux(2),encoder_mux(4)];
    Imux = [motor_mux(5),motor_mux(6)];
    psi = encoder_mux(5);
    Pmux = [motor_mux(1),motor_mux(3)];
end

== matlab function PlanerizerTest07_Flight_Stance/Read Planarizer Leg (Channel 1)/Planarizer Read/Read Planarizer Leg (Chaannel 1)/If Action Subsystem1/bytes -> floats ==
  data: position input; position output; velocity output; velocity input
function [position, velocity] = fcn(position, velocity)

CPR  = 40000;  % [Counts Per Revolution]
F    = 1000;   % [Samples Per Second]

position = position/CPR*(2*pi());
velocity = velocity/CPR*(2*pi())*F;

== matlab function PlanerizerTest07_Flight_Stance/Read Planarizer Leg (Channel 1)/Planarizer Read/Read Planarizer Leg (Chaannel 1)/If Action Subsystem4/bytes -> floats ==
  data: position input; position output; velocity output; velocity input
function [position, velocity] = fcn(position, velocity)

CPR  = 40000;  % [Counts Per Revolution]
F    = 1000;   % [Samples Per Second]

position = position/CPR*(2*pi());
velocity = velocity/CPR*(2*pi())*F;

== matlab function PlanerizerTest07_Flight_Stance/ID2 Write Knee Data/floats -> bytes ==
  data: position input; b output uint8 size=8; velocity input; K_p input; K_d input; T_ff input
function b = fcn(position, velocity, K_p, K_d, T_ff)

P_MIN  =-95.5;  % [rad]
P_MAX  = 95.5;  % [rad]
V_MIN  =-45;    % [rad/s] 30 to 45
V_MAX  = 45;    % [rad/s]
KP_MIN = 0;     % [Nm/rad]
KP_MAX = 500;   % [Nm/rad]
KD_MIN = 0;     % [Nm*s/rad
KD_MAX = 5;     % [Nm*s/rad
T_MIN  =-18;    % [Nm]
T_MAX  = 18;    % [Nm]

position = floor((max(min(position,P_MAX) ,P_MIN)  - P_MIN )*65535/(P_MAX  - P_MIN));
velocity = floor((max(min(velocity,V_MAX) ,V_MIN)  - V_MIN )*4095 /(V_MAX  - V_MIN));
K_p      = floor((max(min(K_p     ,KP_MAX),KP_MIN) - KP_MIN)*4095 /(KP_MAX - KP_MIN));
K_d      = floor((max(min(K_d     ,V_MAX) ,V_MIN)  - KD_MIN)*4095 /(KD_MAX - KD_MIN));
T_ff     = floor((max(min(T_ff    ,V_MAX) ,V_MIN)  - T_MIN )*4095 /(T_MAX  - T_MIN));

p  = dec2bin(position);
p  = [repmat('0', 1, 16-length(p)),p];
v  = dec2bin(velocity);
v  = [repmat('0', 1, 12-length(v)),v];
kp = dec2bin(K_p);
kp  = [repmat('0', 1, 12-length(kp)),kp];
kd = dec2bin(K_d);
kd  = [repmat('0', 1, 12-length(kd)),kd];
t  = dec2bin(T_ff);
t  = [repmat('0', 1, 12-length(t)),t];

B = repmat('0', 8, 8);

B(1,:) = p(1:8);
B(2,:) = p(9:16);
B(3,:) = v(1:8);
B(4,:) = [v(9:12),kp(1:4)];
B(5,:) = kp(5:12);
B(6,:) = kd(1:8);
B(7,:) = [kd(9:12),t(1:4)];
B(8,:) = t(5:12);

B  = bin2dec(B);

b = uint8(B);
